simulink model "problem_6_2"  (R2018b)
settings: Solver=VariableStepAuto  StartTime=0.0  StopTime=15  RelTol=1e-3
values from neighbouring files (symbols this model uses):
  gamma1 = 1    [parameters.m]
  gamma2 = 1    [parameters.m]
  gamma3 = 1    [parameters.m]
settings Model: Creator=cale  LastModifiedBy=cale

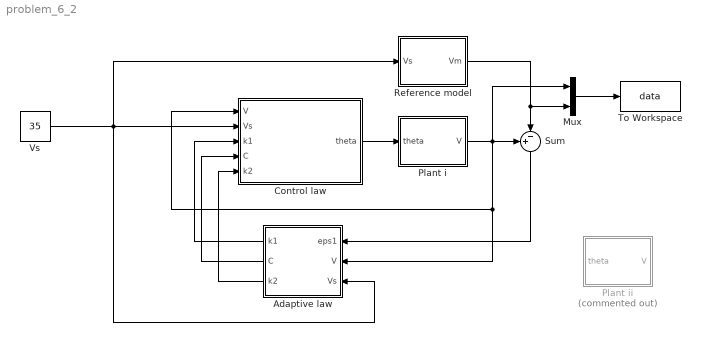
== system problem_6_2 ==
  Adaptive law : Subsystem
  Control law : Subsystem
  Mux : Mux  Inputs=2
  Plant i : Subsystem
  Plant ii : Subsystem  Commented=on
  Reference model : Subsystem
  Sum : Sum  Inputs=+-|
  To Workspace : ToWorkspace  VariableName=data  SaveFormat=Timeseries  SampleTime=-1
  Vs : Constant  Value=35
  wires:
  Plant i/1(V) -> Mux/1, Control law/1(V), Adaptive law/2(V), Sum/1
  Reference model/1(Vm) -> Sum/2, Mux/2
  Control law/1(theta) -> Plant i/1(theta)
  Sum/1 -> Adaptive law/1(eps1)
  Adaptive law/1(k1) -> Control law/3(k1)
  Adaptive law/2(C) -> Control law/4(C)
  Adaptive law/3(k2) -> Control law/5(k2)
  Vs/1 -> Adaptive law/3(Vs), Reference model/1(Vs), Control law/2(Vs)
  Mux/1 -> To Workspace/1

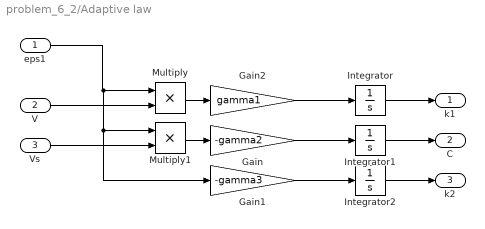
== system problem_6_2/Adaptive law ==
  eps1 : Inport
  V : Inport  Port=2
  Vs : Inport  Port=3
  Gain : Gain  Gain=-gamma2
  Gain1 : Gain  Gain=-gamma3
  Gain2 : Gain  Gain=gamma1
  Integrator : Integrator
  Integrator1 : Integrator
  Integrator2 : Integrator
  Multiply : Product
  Multiply1 : Product
  k1 : Outport
  C : Outport  Port=2
  k2 : Outport  Port=3
  wires:
  Gain/1 -> Integrator1/1
  Gain1/1 -> Integrator2/1
  Gain2/1 -> Integrator/1
  Multiply/1 -> Gain2/1
  eps1/1 -> Gain1/1, Multiply1/1, Multiply/1
  V/1 -> Multiply/2
  Multiply1/1 -> Gain/1
  Vs/1 -> Multiply1/2
  Integrator/1 -> k1/1
  Integrator1/1 -> C/1
  Integrator2/1 -> k2/1

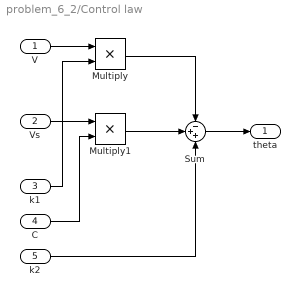
== system problem_6_2/Control law ==
  V : Inport
  Vs : Inport  Port=2
  k1 : Inport  Port=3
  C : Inport  Port=4
  k2 : Inport  Port=5
  Multiply : Product
  Multiply1 : Product
  Sum : Sum  Inputs=-++
  theta : Outport
  wires:
  V/1 -> Multiply/1
  Vs/1 -> Multiply1/1
  Sum/1 -> theta/1
  Multiply1/1 -> Sum/2
  Multiply/1 -> Sum/1
  k1/1 -> Multiply/2
  C/1 -> Multiply1/2
  k2/1 -> Sum/3

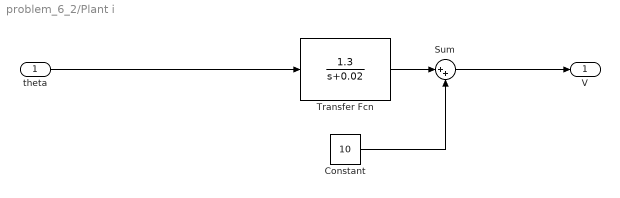
== system problem_6_2/Plant i ==
  theta : Inport
  Constant : Constant  Value=10
  Sum : Sum  Inputs=|++
  Transfer Fcn : TransferFcn  Numerator=[1.3]  Denominator=[1 0.02]
  V : Outport
  wires:
  Transfer Fcn/1 -> Sum/1
  Constant/1 -> Sum/2
  Sum/1 -> V/1
  theta/1 -> Transfer Fcn/1

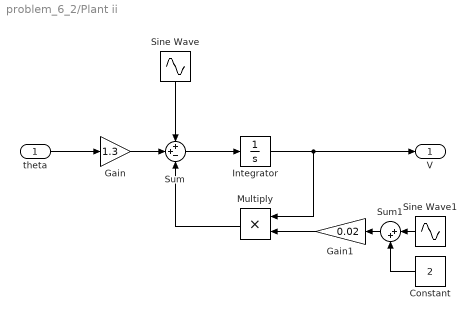
== system problem_6_2/Plant ii ==
  theta : Inport
  Constant : Constant  Value=2
  Gain : Gain  Gain=1.3
  Gain1 : Gain  Gain=0.02
  Integrator : Integrator
  Multiply : Product
  Sine Wave : Sin  Amplitude=10  Frequency=0.02  SampleTime=0
  Sine Wave1 : Sin  Frequency=0.01  SampleTime=0
  Sum : Sum  Inputs=++-
  Sum1 : Sum  Inputs=|++
  V : Outport
  wires:
  Sum/1 -> Integrator/1
  theta/1 -> Gain/1
  Integrator/1 -> Multiply/1, V/1
  Sine Wave/1 -> Sum/1
  Multiply/1 -> Sum/3
  Gain/1 -> Sum/2
  Sine Wave1/1 -> Sum1/1
  Constant/1 -> Sum1/2
  Sum1/1 -> Gain1/1
  Gain1/1 -> Multiply/2

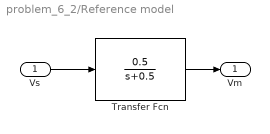
== system problem_6_2/Reference model ==
  Vs : Inport
  Transfer Fcn : TransferFcn  Numerator=[0.5]  Denominator=[1 0.5]
  Vm : Outport
  wires:
  Transfer Fcn/1 -> Vm/1
  Vs/1 -> Transfer Fcn/1
